simulink model "Lab5"  (R2018a)
settings: Solver=VariableStepAuto  StartTime=0.0  StopTime=10.0  RelTol=1e-3
libraries: dsparch4 x4
settings Model: Creator=Hp  LastModifiedBy=Hp

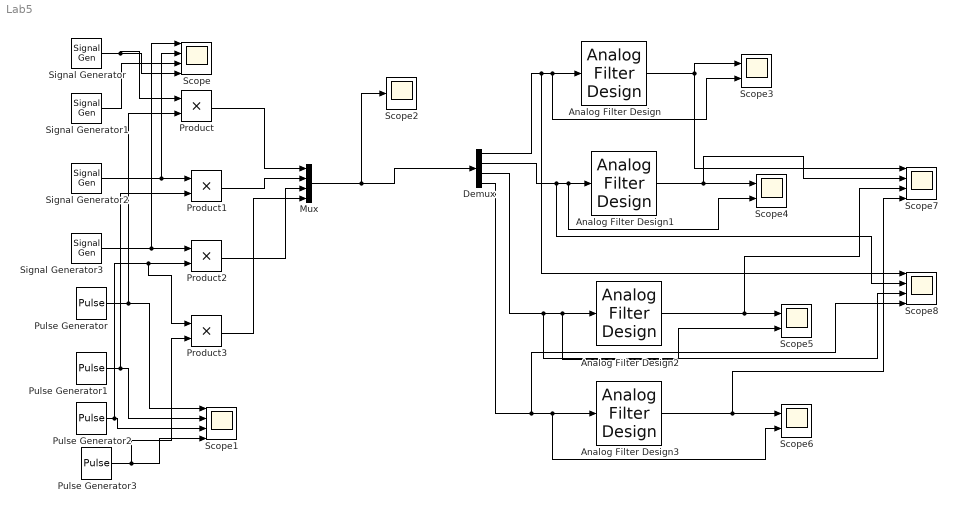
== system Lab5 ==
  Analog Filter Design : dsparch4/Analog Filter Design  method=Butterworth  filttype=Lowpass  N=8  Wlo=2*pi  Whi=80  Rp=2  Rs=40
  Analog Filter Design1 : dsparch4/Analog Filter Design  method=Butterworth  filttype=Lowpass  N=8  Wlo=4*pi  Whi=80  Rp=2  Rs=40
  Analog Filter Design2 : dsparch4/Analog Filter Design  method=Butterworth  filttype=Lowpass  N=8  Wlo=6*pi  Whi=80  Rp=2  Rs=40
  Analog Filter Design3 : dsparch4/Analog Filter Design  method=Butterworth  filttype=Lowpass  N=8  Wlo=8*pi  Whi=80  Rp=2  Rs=40
  Demux : Demux
  Mux : Mux
  Product{,1..3} (4 alike) : Product
  Pulse Generator : DiscretePulseGenerator  PulseType=Time based  Amplitude=0.1  Period=0.1  PulseWidth=5
  Pulse Generator1 : DiscretePulseGenerator  PulseType=Time based  Amplitude=0.2  Period=0.1  PulseWidth=5
  Pulse Generator2 : DiscretePulseGenerator  PulseType=Time based  Amplitude=0.3  Period=0.1  PulseWidth=5
  Pulse Generator3 : DiscretePulseGenerator  PulseType=Time based  Amplitude=0.4  Period=0.1  PulseWidth=5
  Scope{,1,7..8} (4 alike) : Scope  NumInputPorts=4
  Scope2 : Scope
  Scope{3..6} (4 alike) : Scope  NumInputPorts=2
  Signal Generator : SignalGenerator  Amplitude=2*pi  Units=rad/sec
  Signal Generator1 : SignalGenerator  Amplitude=4*pi  Units=rad/sec
  Signal Generator2 : SignalGenerator  Amplitude=6*pi  Units=rad/sec
  Signal Generator3 : SignalGenerator  Amplitude=8*pi  Units=rad/sec
  wires:
  Signal Generator/1 -> Product/1, Scope/4
  Signal Generator1/1 -> Scope/3
  Signal Generator2/1 -> Product1/1, Scope/2
  Signal Generator3/1 -> Product2/1, Scope/1
  Pulse Generator/1 -> Product/2, Scope1/1
  Pulse Generator1/1 -> Product1/2, Scope1/2
  Pulse Generator2/1 -> Product3/1, Product2/2, Scope1/3
  Pulse Generator3/1 -> Product3/2, Scope1/4
  Product/1 -> Mux/1
  Product1/1 -> Mux/2
  Product2/1 -> Mux/3
  Product3/1 -> Mux/4
  Mux/1 -> Scope2/1, Demux/1
  Demux/1 -> Scope8/1, Scope3/2, Analog Filter Design/1
  Demux/2 -> Scope8/2, Scope4/2, Analog Filter Design1/1
  Demux/3 -> Scope8/3, Scope5/2, Analog Filter Design2/1
  Demux/4 -> Scope8/4, Scope6/2, Analog Filter Design3/1
  Analog Filter Design/1 -> Scope7/1, Scope3/1
  Analog Filter Design1/1 -> Scope7/2, Scope4/1
  Analog Filter Design2/1 -> Scope7/3, Scope5/1
  Analog Filter Design3/1 -> Scope7/4, Scope6/1
